simulink model "Aufgabe_1_6"  (R2016b)
settings: Solver=VariableStepAuto  StartTime=0.0  StopTime=0.02  RelTol=1e-3
values from neighbouring files (symbols this model uses):
  a = 0.4    [aufgabe6.m]    (also in cds_matlab_intro_part1.m = 1; test_sfunc_m.m = block.DialogPrm(1).Data)
  c = [0, K]    [Esys_Parameter.m]    (also in aufgabe1.m = 1; aufgabe2.m = 1; aufgabe6.m = 0.5; aufgabe7.m = 1)
  T1 = 10^(-3)    (= 0.001)    [aufgabe6.m]
  Ta = 0.05    [aufgabe1.m]    (also in aufgabe2.m; aufgabe3.m; aufgabe6.m = 1e-06; aufgabe7.m)
libraries: cstblocks x1
settings Model: Creator=M  LastModifiedBy=M
settings SolverCC: AlgebraicLoopSolver=LineSearch

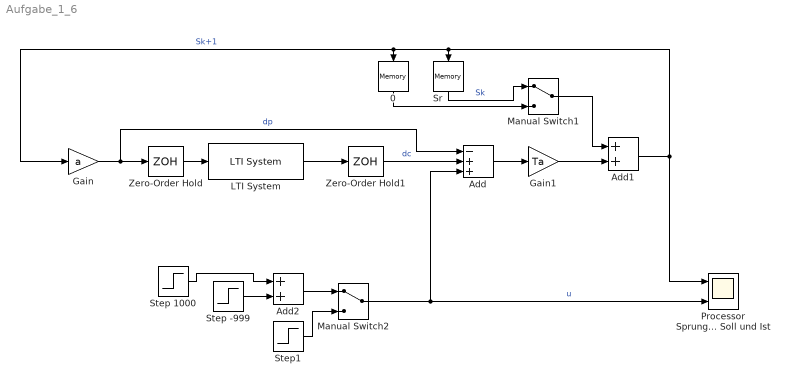
== system Aufgabe_1_6 ==
  0 : Memory
  Add : Sum  Inputs=-++
  Add1 : Sum
  Add2 : Sum
  Gain : Gain  Gain=a
  Gain1 : Gain  Gain=Ta
  LTI System : cstblocks/LTI System  sys=tf(c,[T1 1])  IC=[]
  Manual Switch1 : ManualSwitch
  Manual Switch2 : ManualSwitch
  Processor Sprungantwort Soll und Ist : Scope  NumInputPorts=3
  Sr : Memory  X0=5
  "Step -999 " : Step  Time=0.015  After=-999  SampleTime=Ta
  "Step 1000 " : Step  Time=0.01  Before=1  After=1000  SampleTime=Ta
  Step1 : Step  Time=0  SampleTime=0
  Zero-Order Hold : ZeroOrderHold  SampleTime=Ta
  Zero-Order Hold1 : ZeroOrderHold  SampleTime=Ta
  wires:
  Manual Switch2/1 -> Add/3, Processor Sprungantwort Soll und Ist/3  "u"
  Add/1 -> Gain1/1
  Gain/1 -> Zero-Order Hold/1, Add/1  "dp"
  Gain1/1 -> Add1/2
  Step1/1 -> Manual Switch2/2
  Add2/1 -> Manual Switch2/1
  "Step -999 "/1 -> Add2/2
  "Step 1000 "/1 -> Add2/1
  Add1/1 -> Sr/1, 0/1, Gain/1, Processor Sprungantwort Soll und Ist/1  "Sk+1"
  LTI System/1 -> Zero-Order Hold1/1
  Zero-Order Hold/1 -> LTI System/1
  Zero-Order Hold1/1 -> Add/2  "dc"
  Manual Switch1/1 -> Add1/1
  0/1 -> Manual Switch1/2
  Sr/1 -> Manual Switch1/1  "Sk"
